simulink model "LRC"  (R2022b)
settings: Solver=VariableStepAuto  StartTime=0.0  StopTime=15  RelTol=1e-3
values from neighbouring files (symbols this model uses):
  C = 1    [CircuitoLRC.m]    (also in LRC_simulink_workspace.m = 0.01)
  L = 1    [CircuitoLRC.m]    (also in LRC_simulink_workspace.m)
  R = 1    [CircuitoLRC.m]    (also in LRC_simulink_workspace.m)
  Vi = 2    [LRC_simulink_workspace.m]
settings Model: Creator=giuli  LastModifiedBy=giuli

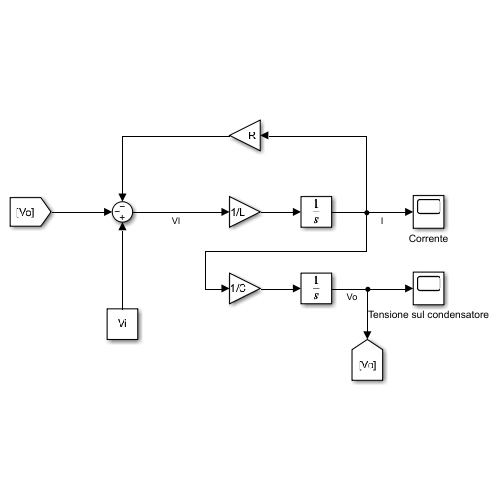
[thumbnail: Simulink's stored preview of the top-level diagram]
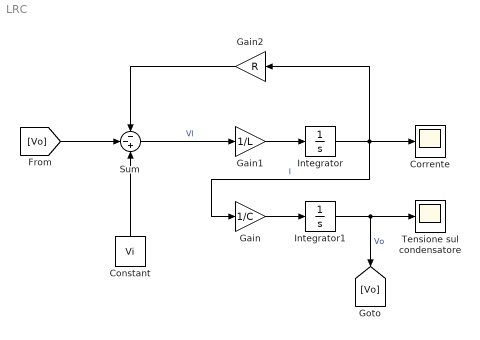
== system LRC ==
  Constant : Constant  Value=Vi
  Corrente : Scope
  Gain : Gain  Gain=1/C
  Gain1 : Gain  Gain=1/L
  Gain2 : Gain  Gain=R
  Integrator : Integrator
  Integrator1 : Integrator
  Sum : Sum  Inputs=--+
  Tensione sul condensatore : Scope
  wires:
  Integrator/1 -> Gain/1, Gain2/1, Corrente/1  "I"
  Integrator1/1 -> Tensione sul condensatore/1, [Vo]  "Vo"
  Gain1/1 -> Integrator/1
  Sum/1 -> Gain1/1  "Vl"
  [Vo] -> Sum/2
  Constant/1 -> Sum/3
  Gain2/1 -> Sum/1
  Gain/1 -> Integrator1/1
